simulink model "life_flow"  (R2018b)
settings: Solver=VariableStepAuto  StartTime=0.0  StopTime=10.0  RelTol=1e-3
settings Model: Creator=108  LastModifiedBy=108

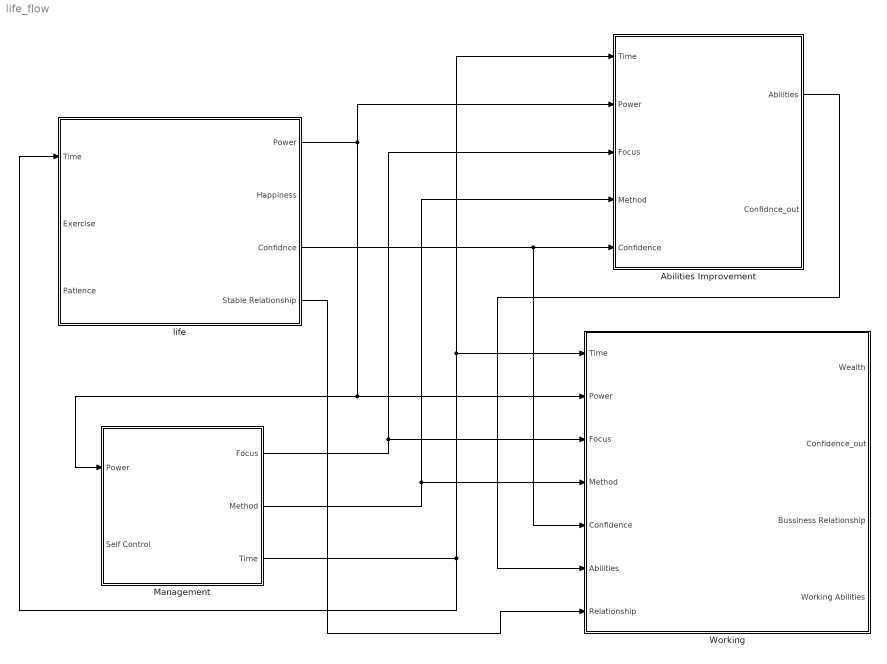
== system life_flow ==
  Abilities Improvement : Subsystem
  Management : Subsystem
  Working : Subsystem
  life : Subsystem
  wires:
  life/1(Power) -> Abilities Improvement/2(Power), Management/1(Power), Working/2(Power)
  life/3(Confidnce) -> Abilities Improvement/5(Confidence), Working/5(Confidence)
  Management/1(Focus) -> Working/3(Focus), Abilities Improvement/3(Focus)
  Management/3(Time) -> life/1(Time), Working/1(Time), Abilities Improvement/1(Time)
  Management/2(Method) -> Working/4(Method), Abilities Improvement/4(Method)
  Abilities Improvement/1(Abilities) -> Working/6(Abilities)
  life/4(Stable Relationship) -> Working/7(Relationship)

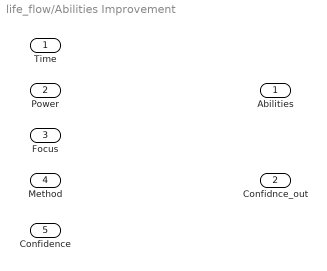
== system life_flow/Abilities Improvement ==
  Time : Inport
  Power : Inport  Port=2
  Focus : Inport  Port=3
  Method : Inport  Port=4
  Confidence : Inport  Port=5
  Abilities : Outport
  Confidnce_out : Outport  Port=2

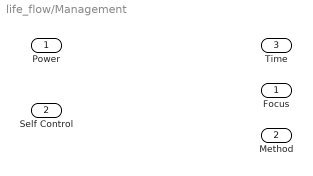
== system life_flow/Management ==
  Power : Inport
  Self Control : Inport  Port=2
  Focus : Outport
  Method : Outport  Port=2
  Time : Outport  Port=3

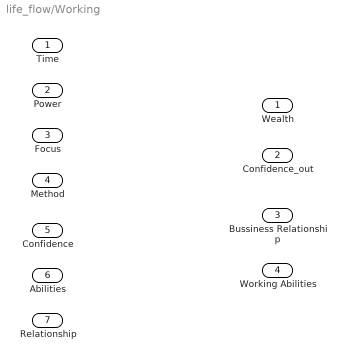
== system life_flow/Working ==
  Time : Inport
  Power : Inport  Port=2
  Focus : Inport  Port=3
  Method : Inport  Port=4
  Confidence : Inport  Port=5
  Abilities : Inport  Port=6
  Relationship : Inport  Port=7
  Wealth : Outport
  Confidence_out : Outport  Port=2
  Bussiness Relationship : Outport  Port=3
  Working Abilities : Outport  Port=4

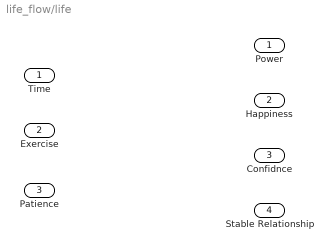
== system life_flow/life ==
  Time : Inport
  Exercise : Inport  Port=2
  Patience : Inport  Port=3
  Power : Outport
  Happiness : Outport  Port=2
  Confidnce : Outport  Port=3
  Stable Relationship : Outport  Port=4
